simulink model "pruebas"  (R2018b)
settings: Solver=VariableStepAuto  StartTime=0.0  StopTime=10.0  RelTol=1e-3
settings Model: Creator=kurama  LastModifiedBy=kurama

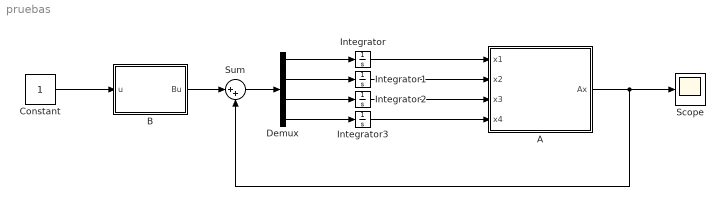
== system pruebas ==
  A : MATLAB Function  TreatAsAtomicUnit=on
  "B " : MATLAB Function  TreatAsAtomicUnit=on
  Constant : Constant
  Demux : Demux
  Integrator : Integrator  InitialCondition=1
  Integrator1 : Integrator  InitialCondition=-1
  Integrator2 : Integrator
  Integrator3 : Integrator  InitialCondition=2
  Scope : Scope
  Sum : Sum  Inputs=|++
  wires:
  "B "/1(Bu) -> Sum/1
  A/1(Ax) -> Scope/1, Sum/2
  Integrator/1 -> A/1(x1)
  Integrator1/1 -> A/2(x2)
  Integrator2/1 -> A/3(x3)
  Integrator3/1 -> A/4(x4)
  Sum/1 -> Demux/1
  Demux/1 -> Integrator/1
  Demux/2 -> Integrator1/1
  Demux/3 -> Integrator2/1
  Demux/4 -> Integrator3/1
  Constant/1 -> "B "/1(u)

== matlab function pruebas/B  ==
  data: u input; Bu output
function Bu = fcn(u)

u = u * [1;
         1];

B = [-1, -4;
      1,  6;
     -1, -11;
      1,  7];
  
% B = [-1;
%       1;
%      -1;
%       1];

Bu = B*u;

== matlab function pruebas/A ==
  data: x1 input; Ax output; x2 input; x3 input; x4 input
function Ax = fcn(x1, x2, x3, x4)

x = [x1;
     x2;
     x3;
     x4];

A = [ 2, -11,  12,  31;
     -3,  13, -11, -33;
      4, -25,  14,  51;
     -3,  16, -11, -36];

Ax = A*x;
